simulink model "gm_MATE_HDLsolver_myFirstCircuit"  (R2024b)
settings: Solver=FixedStepDiscrete  StartTime=0.0  StopTime=0.05  FixedStep=6.02409638554217e-09  MaxStep=100e-6  RelTol=1e-4
PostLoadFcn:
  | Ts=1e-6; nb_sw=3; nb_lc=2;nb_r=1;nb_src=1; nb_out=3; rL=1.2;rC=100;L=1e-3; C=1e-5; LpejoSw=1e-6;h=Ts; MAX_INPUTS=16;
  | MAX_OUTPUTS=16;
  | MAX_SWITCHES=8;
  | MAX_INPUTS=16;
InitFcn:
  | Ts=1e-6; nb_sw=3; nb_lc=2;nb_r=1;nb_src=1; nb_out=3; rL=1.2;rC=100;L=1e-3; C=1e-5; LpejoSw=1e-6;h=Ts; MAX_INPUTS=16;
  | MAX_OUTPUTS=16;
  | MAX_SWITCHES=8;
  | MAX_INPUTS=16;
undefined symbols (not defined in the file or in its folder): MATE_SOC
libraries: fl_lib x31, nesl_utility x13, hdlmdlgenlib x10, simetranss x5, simulink x4, hdlsllib x3, ee_lib x2, eeGeneralControl x1
(part 5 of 8)

== system gm_MATE_HDLsolver_myFirstCircuit/ForFPGA/Dot Product79 ==
  In1 : Inport
  In2 : Inport  Port=2
  Dot Product79 : Sum  OutDataTypeStr=single  SampleTime=6.02409638554217e-09
  Dot Product79_pd1 : Delay  DelayLength=6
  Out1 : Outport
  wires:
  In1/1 -> Dot Product79/1
  In2/1 -> Dot Product79/2
  Dot Product79/1 -> Dot Product79_pd1/1
  Dot Product79_pd1/1 -> Out1/1

== system gm_MATE_HDLsolver_myFirstCircuit/ForFPGA/Dot Product8 ==
  In1 : Inport
  In2 : Inport  Port=2
  Dot Product8 : Sum  OutDataTypeStr=single  SampleTime=6.02409638554217e-09
  Dot Product8_pd1 : Delay  DelayLength=6
  Out1 : Outport
  wires:
  In1/1 -> Dot Product8/1
  In2/1 -> Dot Product8/2
  Dot Product8/1 -> Dot Product8_pd1/1
  Dot Product8_pd1/1 -> Out1/1

== system gm_MATE_HDLsolver_myFirstCircuit/ForFPGA/Dot Product81 ==
  In1 : Inport
  In2 : Inport  Port=2
  Dot Product81 : Sum  OutDataTypeStr=single  SampleTime=6.02409638554217e-09
  Dot Product81_pd1 : Delay  DelayLength=6
  Out1 : Outport
  wires:
  In1/1 -> Dot Product81/1
  In2/1 -> Dot Product81/2
  Dot Product81/1 -> Dot Product81_pd1/1
  Dot Product81_pd1/1 -> Out1/1

== system gm_MATE_HDLsolver_myFirstCircuit/ForFPGA/Dot Product810 ==
  In1 : Inport
  In2 : Inport  Port=2
  Dot Product810 : Sum  OutDataTypeStr=single  SampleTime=6.02409638554217e-09
  Dot Product810_pd1 : Delay  DelayLength=6
  Out1 : Outport
  wires:
  In1/1 -> Dot Product810/1
  In2/1 -> Dot Product810/2
  Dot Product810/1 -> Dot Product810_pd1/1
  Dot Product810_pd1/1 -> Out1/1

== system gm_MATE_HDLsolver_myFirstCircuit/ForFPGA/Dot Product811 ==
  In1 : Inport
  In2 : Inport  Port=2
  Dot Product811 : Sum  OutDataTypeStr=single  SampleTime=6.02409638554217e-09
  Dot Product811_pd1 : Delay  DelayLength=6
  Out1 : Outport
  wires:
  In1/1 -> Dot Product811/1
  In2/1 -> Dot Product811/2
  Dot Product811/1 -> Dot Product811_pd1/1
  Dot Product811_pd1/1 -> Out1/1

== system gm_MATE_HDLsolver_myFirstCircuit/ForFPGA/Dot Product812 ==
  In1 : Inport
  In2 : Inport  Port=2
  Dot Product812 : Sum  OutDataTypeStr=single  SampleTime=6.02409638554217e-09
  Dot Product812_pd1 : Delay  DelayLength=6
  Out1 : Outport
  wires:
  In1/1 -> Dot Product812/1
  In2/1 -> Dot Product812/2
  Dot Product812/1 -> Dot Product812_pd1/1
  Dot Product812_pd1/1 -> Out1/1

== system gm_MATE_HDLsolver_myFirstCircuit/ForFPGA/Dot Product813 ==
  In1 : Inport
  In2 : Inport  Port=2
  Dot Product813 : Sum  OutDataTypeStr=single  SampleTime=6.02409638554217e-09
  Dot Product813_pd1 : Delay  DelayLength=6
  Out1 : Outport
  wires:
  In1/1 -> Dot Product813/1
  In2/1 -> Dot Product813/2
  Dot Product813/1 -> Dot Product813_pd1/1
  Dot Product813_pd1/1 -> Out1/1

== system gm_MATE_HDLsolver_myFirstCircuit/ForFPGA/Dot Product814 ==
  In1 : Inport
  In2 : Inport  Port=2
  Dot Product814 : Sum  OutDataTypeStr=single  SampleTime=6.02409638554217e-09
  Dot Product814_pd1 : Delay  DelayLength=6
  Out1 : Outport
  wires:
  In1/1 -> Dot Product814/1
  In2/1 -> Dot Product814/2
  Dot Product814/1 -> Dot Product814_pd1/1
  Dot Product814_pd1/1 -> Out1/1

== system gm_MATE_HDLsolver_myFirstCircuit/ForFPGA/Dot Product815 ==
  In1 : Inport
  In2 : Inport  Port=2
  Dot Product815 : Sum  OutDataTypeStr=single  SampleTime=6.02409638554217e-09
  Dot Product815_pd1 : Delay  DelayLength=6
  Out1 : Outport
  wires:
  In1/1 -> Dot Product815/1
  In2/1 -> Dot Product815/2
  Dot Product815/1 -> Dot Product815_pd1/1
  Dot Product815_pd1/1 -> Out1/1

== system gm_MATE_HDLsolver_myFirstCircuit/ForFPGA/Dot Product82 ==
  In1 : Inport
  In2 : Inport  Port=2
  Dot Product82 : Sum  OutDataTypeStr=single  SampleTime=6.02409638554217e-09
  Dot Product82_pd1 : Delay  DelayLength=6
  Out1 : Outport
  wires:
  In1/1 -> Dot Product82/1
  In2/1 -> Dot Product82/2
  Dot Product82/1 -> Dot Product82_pd1/1
  Dot Product82_pd1/1 -> Out1/1

== system gm_MATE_HDLsolver_myFirstCircuit/ForFPGA/Dot Product83 ==
  In1 : Inport
  In2 : Inport  Port=2
  Dot Product83 : Sum  OutDataTypeStr=single  SampleTime=6.02409638554217e-09
  Dot Product83_pd1 : Delay  DelayLength=6
  Out1 : Outport
  wires:
  In1/1 -> Dot Product83/1
  In2/1 -> Dot Product83/2
  Dot Product83/1 -> Dot Product83_pd1/1
  Dot Product83_pd1/1 -> Out1/1

== system gm_MATE_HDLsolver_myFirstCircuit/ForFPGA/Dot Product84 ==
  In1 : Inport
  In2 : Inport  Port=2
  Dot Product84 : Sum  OutDataTypeStr=single  SampleTime=6.02409638554217e-09
  Dot Product84_pd1 : Delay  DelayLength=6
  Out1 : Outport
  wires:
  In1/1 -> Dot Product84/1
  In2/1 -> Dot Product84/2
  Dot Product84/1 -> Dot Product84_pd1/1
  Dot Product84_pd1/1 -> Out1/1

== system gm_MATE_HDLsolver_myFirstCircuit/ForFPGA/Dot Product85 ==
  In1 : Inport
  In2 : Inport  Port=2
  Dot Product85 : Sum  OutDataTypeStr=single  SampleTime=6.02409638554217e-09
  Dot Product85_pd1 : Delay  DelayLength=6
  Out1 : Outport
  wires:
  In1/1 -> Dot Product85/1
  In2/1 -> Dot Product85/2
  Dot Product85/1 -> Dot Product85_pd1/1
  Dot Product85_pd1/1 -> Out1/1

== system gm_MATE_HDLsolver_myFirstCircuit/ForFPGA/Dot Product86 ==
  In1 : Inport
  In2 : Inport  Port=2
  Dot Product86 : Sum  OutDataTypeStr=single  SampleTime=6.02409638554217e-09
  Dot Product86_pd1 : Delay  DelayLength=6
  Out1 : Outport
  wires:
  In1/1 -> Dot Product86/1
  In2/1 -> Dot Product86/2
  Dot Product86/1 -> Dot Product86_pd1/1
  Dot Product86_pd1/1 -> Out1/1

== system gm_MATE_HDLsolver_myFirstCircuit/ForFPGA/Dot Product87 ==
  In1 : Inport
  In2 : Inport  Port=2
  Dot Product87 : Sum  OutDataTypeStr=single  SampleTime=6.02409638554217e-09
  Dot Product87_pd1 : Delay  DelayLength=6
  Out1 : Outport
  wires:
  In1/1 -> Dot Product87/1
  In2/1 -> Dot Product87/2
  Dot Product87/1 -> Dot Product87_pd1/1
  Dot Product87_pd1/1 -> Out1/1

== system gm_MATE_HDLsolver_myFirstCircuit/ForFPGA/Dot Product88 ==
  In1 : Inport
  In2 : Inport  Port=2
  Dot Product88 : Sum  OutDataTypeStr=single  SampleTime=6.02409638554217e-09
  Dot Product88_pd1 : Delay  DelayLength=6
  Out1 : Outport
  wires:
  In1/1 -> Dot Product88/1
  In2/1 -> Dot Product88/2
  Dot Product88/1 -> Dot Product88_pd1/1
  Dot Product88_pd1/1 -> Out1/1

== system gm_MATE_HDLsolver_myFirstCircuit/ForFPGA/Dot Product89 ==
  In1 : Inport
  In2 : Inport  Port=2
  Dot Product89 : Sum  OutDataTypeStr=single  SampleTime=6.02409638554217e-09
  Dot Product89_pd1 : Delay  DelayLength=6
  Out1 : Outport
  wires:
  In1/1 -> Dot Product89/1
  In2/1 -> Dot Product89/2
  Dot Product89/1 -> Dot Product89_pd1/1
  Dot Product89_pd1/1 -> Out1/1

== system gm_MATE_HDLsolver_myFirstCircuit/ForFPGA/Dot Product9 ==
  In1 : Inport
  In2 : Inport  Port=2
  Dot Product9 : Sum  OutDataTypeStr=single  SampleTime=6.02409638554217e-09
  Dot Product9_pd1 : Delay  DelayLength=6
  Out1 : Outport
  wires:
  In1/1 -> Dot Product9/1
  In2/1 -> Dot Product9/2
  Dot Product9/1 -> Dot Product9_pd1/1
  Dot Product9_pd1/1 -> Out1/1

== system gm_MATE_HDLsolver_myFirstCircuit/ForFPGA/Dot Product91 ==
  In1 : Inport
  In2 : Inport  Port=2
  Dot Product91 : Sum  OutDataTypeStr=single  SampleTime=6.02409638554217e-09
  Dot Product91_pd1 : Delay  DelayLength=6
  Out1 : Outport
  wires:
  In1/1 -> Dot Product91/1
  In2/1 -> Dot Product91/2
  Dot Product91/1 -> Dot Product91_pd1/1
  Dot Product91_pd1/1 -> Out1/1

== system gm_MATE_HDLsolver_myFirstCircuit/ForFPGA/Dot Product910 ==
  In1 : Inport
  In2 : Inport  Port=2
  Dot Product910 : Sum  OutDataTypeStr=single  SampleTime=6.02409638554217e-09
  Dot Product910_pd1 : Delay  DelayLength=6
  Out1 : Outport
  wires:
  In1/1 -> Dot Product910/1
  In2/1 -> Dot Product910/2
  Dot Product910/1 -> Dot Product910_pd1/1
  Dot Product910_pd1/1 -> Out1/1

== system gm_MATE_HDLsolver_myFirstCircuit/ForFPGA/Dot Product911 ==
  In1 : Inport
  In2 : Inport  Port=2
  Dot Product911 : Sum  OutDataTypeStr=single  SampleTime=6.02409638554217e-09
  Dot Product911_pd1 : Delay  DelayLength=6
  Out1 : Outport
  wires:
  In1/1 -> Dot Product911/1
  In2/1 -> Dot Product911/2
  Dot Product911/1 -> Dot Product911_pd1/1
  Dot Product911_pd1/1 -> Out1/1

== system gm_MATE_HDLsolver_myFirstCircuit/ForFPGA/Dot Product912 ==
  In1 : Inport
  In2 : Inport  Port=2
  Dot Product912 : Sum  OutDataTypeStr=single  SampleTime=6.02409638554217e-09
  Dot Product912_pd1 : Delay  DelayLength=6
  Out1 : Outport
  wires:
  In1/1 -> Dot Product912/1
  In2/1 -> Dot Product912/2
  Dot Product912/1 -> Dot Product912_pd1/1
  Dot Product912_pd1/1 -> Out1/1

== system gm_MATE_HDLsolver_myFirstCircuit/ForFPGA/Dot Product913 ==
  In1 : Inport
  In2 : Inport  Port=2
  Dot Product913 : Sum  OutDataTypeStr=single  SampleTime=6.02409638554217e-09
  Dot Product913_pd1 : Delay  DelayLength=6
  Out1 : Outport
  wires:
  In1/1 -> Dot Product913/1
  In2/1 -> Dot Product913/2
  Dot Product913/1 -> Dot Product913_pd1/1
  Dot Product913_pd1/1 -> Out1/1

== system gm_MATE_HDLsolver_myFirstCircuit/ForFPGA/Dot Product914 ==
  In1 : Inport
  In2 : Inport  Port=2
  Dot Product914 : Sum  OutDataTypeStr=single  SampleTime=6.02409638554217e-09
  Dot Product914_pd1 : Delay  DelayLength=6
  Out1 : Outport
  wires:
  In1/1 -> Dot Product914/1
  In2/1 -> Dot Product914/2
  Dot Product914/1 -> Dot Product914_pd1/1
  Dot Product914_pd1/1 -> Out1/1

== system gm_MATE_HDLsolver_myFirstCircuit/ForFPGA/Dot Product915 ==
  In1 : Inport
  In2 : Inport  Port=2
  Dot Product915 : Sum  OutDataTypeStr=single  SampleTime=6.02409638554217e-09
  Dot Product915_pd1 : Delay  DelayLength=6
  Out1 : Outport
  wires:
  In1/1 -> Dot Product915/1
  In2/1 -> Dot Product915/2
  Dot Product915/1 -> Dot Product915_pd1/1
  Dot Product915_pd1/1 -> Out1/1

== system gm_MATE_HDLsolver_myFirstCircuit/ForFPGA/Dot Product92 ==
  In1 : Inport
  In2 : Inport  Port=2
  Dot Product92 : Sum  OutDataTypeStr=single  SampleTime=6.02409638554217e-09
  Dot Product92_pd1 : Delay  DelayLength=6
  Out1 : Outport
  wires:
  In1/1 -> Dot Product92/1
  In2/1 -> Dot Product92/2
  Dot Product92/1 -> Dot Product92_pd1/1
  Dot Product92_pd1/1 -> Out1/1

== system gm_MATE_HDLsolver_myFirstCircuit/ForFPGA/Dot Product93 ==
  In1 : Inport
  In2 : Inport  Port=2
  Dot Product93 : Sum  OutDataTypeStr=single  SampleTime=6.02409638554217e-09
  Dot Product93_pd1 : Delay  DelayLength=6
  Out1 : Outport
  wires:
  In1/1 -> Dot Product93/1
  In2/1 -> Dot Product93/2
  Dot Product93/1 -> Dot Product93_pd1/1
  Dot Product93_pd1/1 -> Out1/1

== system gm_MATE_HDLsolver_myFirstCircuit/ForFPGA/Dot Product94 ==
  In1 : Inport
  In2 : Inport  Port=2
  Dot Product94 : Sum  OutDataTypeStr=single  SampleTime=6.02409638554217e-09
  Dot Product94_pd1 : Delay  DelayLength=6
  Out1 : Outport
  wires:
  In1/1 -> Dot Product94/1
  In2/1 -> Dot Product94/2
  Dot Product94/1 -> Dot Product94_pd1/1
  Dot Product94_pd1/1 -> Out1/1

== system gm_MATE_HDLsolver_myFirstCircuit/ForFPGA/Dot Product95 ==
  In1 : Inport
  In2 : Inport  Port=2
  Dot Product95 : Sum  OutDataTypeStr=single  SampleTime=6.02409638554217e-09
  Dot Product95_pd1 : Delay  DelayLength=6
  Out1 : Outport
  wires:
  In1/1 -> Dot Product95/1
  In2/1 -> Dot Product95/2
  Dot Product95/1 -> Dot Product95_pd1/1
  Dot Product95_pd1/1 -> Out1/1

== system gm_MATE_HDLsolver_myFirstCircuit/ForFPGA/Dot Product96 ==
  In1 : Inport
  In2 : Inport  Port=2
  Dot Product96 : Sum  OutDataTypeStr=single  SampleTime=6.02409638554217e-09
  Dot Product96_pd1 : Delay  DelayLength=6
  Out1 : Outport
  wires:
  In1/1 -> Dot Product96/1
  In2/1 -> Dot Product96/2
  Dot Product96/1 -> Dot Product96_pd1/1
  Dot Product96_pd1/1 -> Out1/1

== system gm_MATE_HDLsolver_myFirstCircuit/ForFPGA/Dot Product97 ==
  In1 : Inport
  In2 : Inport  Port=2
  Dot Product97 : Sum  OutDataTypeStr=single  SampleTime=6.02409638554217e-09
  Dot Product97_pd1 : Delay  DelayLength=6
  Out1 : Outport
  wires:
  In1/1 -> Dot Product97/1
  In2/1 -> Dot Product97/2
  Dot Product97/1 -> Dot Product97_pd1/1
  Dot Product97_pd1/1 -> Out1/1

== system gm_MATE_HDLsolver_myFirstCircuit/ForFPGA/Dot Product98 ==
  In1 : Inport
  In2 : Inport  Port=2
  Dot Product98 : Sum  OutDataTypeStr=single  SampleTime=6.02409638554217e-09
  Dot Product98_pd1 : Delay  DelayLength=6
  Out1 : Outport
  wires:
  In1/1 -> Dot Product98/1
  In2/1 -> Dot Product98/2
  Dot Product98/1 -> Dot Product98_pd1/1
  Dot Product98_pd1/1 -> Out1/1

== system gm_MATE_HDLsolver_myFirstCircuit/ForFPGA/Dot Product99 ==
  In1 : Inport
  In2 : Inport  Port=2
  Dot Product99 : Sum  OutDataTypeStr=single  SampleTime=6.02409638554217e-09
  Dot Product99_pd1 : Delay  DelayLength=6
  Out1 : Outport
  wires:
  In1/1 -> Dot Product99/1
  In2/1 -> Dot Product99/2
  Dot Product99/1 -> Dot Product99_pd1/1
  Dot Product99_pd1/1 -> Out1/1

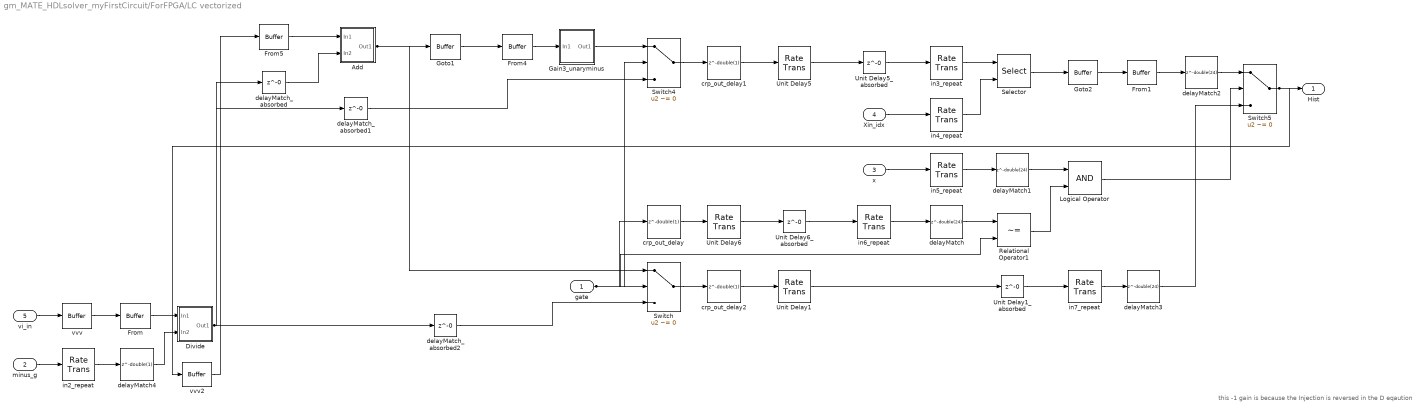
== system gm_MATE_HDLsolver_myFirstCircuit/ForFPGA/LC vectorized ==
  note: this -1 gain is because the Injection is reversed in the D eqaution
  gate : Inport  OutDataTypeStr=boolean  PortDimensions=[5]  SampleTime=6.02409638554217e-09
  minus_g : Inport  Port=2  OutDataTypeStr=single  PortDimensions=[5]  SampleTime=1e-06
  x : Inport  Port=3  OutDataTypeStr=boolean  PortDimensions=[5]  SampleTime=1e-06
  Xin_idx : Inport  Port=4  OutDataTypeStr=uint16  PortDimensions=[5]  SampleTime=1e-06
  vi_in : Inport  Port=5  OutDataTypeStr=single  PortDimensions=[5]  SampleTime=6.02409638554217e-09
  Add : Subsystem
      mask Display: disp('NFP\nadd');
  Divide : Subsystem
      mask Display: disp('NFP\nmul');
  From{,1,4..5} (4 alike) : hdlmdlgenlib/Buffer
  Gain3_unaryminus : Subsystem
      mask Display: disp('NFP\numinus');
  Goto1 : hdlmdlgenlib/Buffer
  Goto2 : hdlmdlgenlib/Buffer
  Logical Operator : Logic  AllPortsSameDT=off  OutDataTypeStr=boolean  SampleTime=6.02409638554217e-09
  Relational Operator1 : RelationalOperator  Operator=~=  OutDataTypeStr=boolean  SampleTime=6.02409638554217e-09  InputSameDT=off
  Selector : Selector  InputPortWidth=5  IndexOptions=Index vector (port)  Indices=double([2 1 3 4 5])  OutputSizes=double(1)
  Switch : Switch  Criteria=u2 ~= 0  Threshold=double(0)  OutDataTypeStr=single  SampleTime=6.02409638554217e-09  SaturateOnIntegerOverflow=off  InputSameDT=off
  Switch4 : Switch  Criteria=u2 ~= 0  Threshold=double(0)  OutDataTypeStr=single  SampleTime=6.02409638554217e-09  SaturateOnIntegerOverflow=off  InputSameDT=off
  Switch5 : Switch  Criteria=u2 ~= 0  Threshold=double(0)  OutDataTypeStr=single  SampleTime=6.02409638554217e-09  SaturateOnIntegerOverflow=off  InputSameDT=off
  Unit Delay1 : RateTransition  InitialCondition=double(0)  OutPortSampleTimeOpt=Multiple of input port sample time  OutPortSampleTimeMultiple=166
  Unit Delay1_absorbed : Delay  DelayLength=0
  Unit Delay5 : RateTransition  InitialCondition=double(0)  OutPortSampleTimeOpt=Multiple of input port sample time  OutPortSampleTimeMultiple=166
  Unit Delay5_absorbed : Delay  DelayLength=0
  Unit Delay6 : RateTransition  InitialCondition=double(0)  OutPortSampleTimeOpt=Multiple of input port sample time  OutPortSampleTimeMultiple=166
  Unit Delay6_absorbed : Delay  DelayLength=0
  crp_out_delay : Delay  DelayLength=double(1)  InitialCondition=0  SampleTime=6.02409638554217e-09
  crp_out_delay1 : Delay  DelayLength=double(1)  InitialCondition=0  SampleTime=6.02409638554217e-09
  crp_out_delay2 : Delay  DelayLength=double(1)  InitialCondition=0  SampleTime=6.02409638554217e-09
  delayMatch{,1..3} (4 alike) : Delay  DelayLength=double(24)  InitialCondition=0  SampleTime=6.02409638554217e-09
  delayMatch4 : Delay  DelayLength=double(1)  InitialCondition=0  SampleTime=6.02409638554217e-09
  delayMatch_absorbed : Delay  DelayLength=0
  delayMatch_absorbed1 : Delay  DelayLength=0
  delayMatch_absorbed2 : Delay  DelayLength=0
  in2_repeat : RateTransition  Integrity=off  Deterministic=off  OutPortSampleTimeOpt=Multiple of input port sample time  OutPortSampleTimeMultiple=1/166
  in3_repeat : RateTransition  Integrity=off  Deterministic=off  OutPortSampleTimeOpt=Multiple of input port sample time  OutPortSampleTimeMultiple=1/166
  in4_repeat : RateTransition  Integrity=off  Deterministic=off  OutPortSampleTimeOpt=Multiple of input port sample time  OutPortSampleTimeMultiple=1/166
  in5_repeat : RateTransition  Integrity=off  Deterministic=off  OutPortSampleTimeOpt=Multiple of input port sample time  OutPortSampleTimeMultiple=1/166
  in6_repeat : RateTransition  Integrity=off  Deterministic=off  OutPortSampleTimeOpt=Multiple of input port sample time  OutPortSampleTimeMultiple=1/166
  in7_repeat : RateTransition  Integrity=off  Deterministic=off  OutPortSampleTimeOpt=Multiple of input port sample time  OutPortSampleTimeMultiple=1/166
  vvv : hdlmdlgenlib/Buffer
  vvv2 : hdlmdlgenlib/Buffer
  Hist : Outport  SampleTime=6.02409638554217e-09
  wires:
  delayMatch4/1 -> Divide/2(In2)
  in7_repeat/1 -> delayMatch3/1
  vi_in/1 -> vvv/1
  Logical Operator/1 -> Switch5/2
  minus_g/1 -> in2_repeat/1
  vvv2/1 -> From5/1
  Unit Delay1/1 -> Unit Delay1_absorbed/1
  in2_repeat/1 -> delayMatch4/1
  delayMatch_absorbed2/1 -> Switch/3
  Divide/1(Out1) -> delayMatch_absorbed1/1, delayMatch_absorbed2/1, delayMatch_absorbed/1
  vvv/1 -> From/1
  From/1 -> Divide/1(In1)
  From5/1 -> Add/1(In1)
  delayMatch_absorbed/1 -> Add/2(In2)
  Add/1(Out1) -> Goto1/1, Switch/1
  crp_out_delay1/1 -> Unit Delay5/1
  delayMatch_absorbed1/1 -> Switch4/3
  Goto1/1 -> From4/1
  From4/1 -> Gain3_unaryminus/1(In1)
  Gain3_unaryminus/1(Out1) -> Switch4/1
  Unit Delay6/1 -> Unit Delay6_absorbed/1
  gate/1 -> Relational Operator1/2, crp_out_delay/1, Switch/2, Switch4/2
  Switch4/1 -> crp_out_delay1/1
  in4_repeat/1 -> Selector/2
  crp_out_delay/1 -> Unit Delay6/1
  Xin_idx/1 -> in4_repeat/1
  Switch/1 -> crp_out_delay2/1
  crp_out_delay2/1 -> Unit Delay1/1
  Unit Delay5/1 -> Unit Delay5_absorbed/1
  Unit Delay1_absorbed/1 -> in7_repeat/1
  Unit Delay6_absorbed/1 -> in6_repeat/1
  Unit Delay5_absorbed/1 -> in3_repeat/1
  Switch5/1 -> Hist/1, vvv2/1
  x/1 -> in5_repeat/1
  in6_repeat/1 -> delayMatch/1
  in3_repeat/1 -> Selector/1
  in5_repeat/1 -> delayMatch1/1
  delayMatch/1 -> Relational Operator1/1
  Selector/1 -> Goto2/1
  delayMatch3/1 -> Switch5/3
  delayMatch1/1 -> Logical Operator/1
  Relational Operator1/1 -> Logical Operator/2
  Goto2/1 -> From1/1
  From1/1 -> delayMatch2/1
  delayMatch2/1 -> Switch5/1

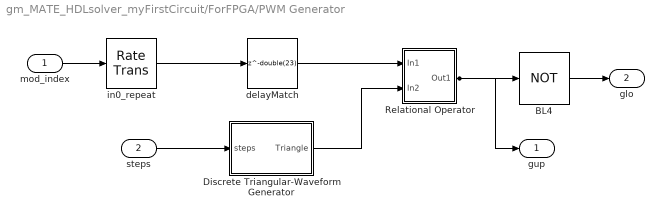
== system gm_MATE_HDLsolver_myFirstCircuit/ForFPGA/PWM Generator ==
  mod_index : Inport  OutDataTypeStr=single  PortDimensions=1  SampleTime=1e-06
  steps : Inport  Port=2  OutDataTypeStr=uint16  PortDimensions=1  SampleTime=1e-06
  BL4 : Logic  Operator=NOT  Inputs=1  AllPortsSameDT=off  OutDataTypeStr=boolean  SampleTime=6.02409638554217e-09
  Discrete Triangular-Waveform Generator : Subsystem
  Relational Operator : Subsystem
      mask Display: disp('NFP\nrelop');
  delayMatch : Delay  DelayLength=double(23)  InitialCondition=0  SampleTime=6.02409638554217e-09
  in0_repeat : RateTransition  Integrity=off  Deterministic=off  OutPortSampleTimeOpt=Multiple of input port sample time  OutPortSampleTimeMultiple=1/166
  gup : Outport  SampleTime=6.02409638554217e-09  VectorParamsAs1DForOutWhenUnconnected=off
  glo : Outport  Port=2  SampleTime=6.02409638554217e-09  VectorParamsAs1DForOutWhenUnconnected=off
  wires:
  Relational Operator/1(Out1) -> gup/1, BL4/1
  mod_index/1 -> in0_repeat/1
  delayMatch/1 -> Relational Operator/1(In1)
  in0_repeat/1 -> delayMatch/1
  steps/1 -> Discrete Triangular-Waveform Generator/1(steps)
  Discrete Triangular-Waveform Generator/1(Triangle) -> Relational Operator/2(In2)
  BL4/1 -> glo/1

== system gm_MATE_HDLsolver_myFirstCircuit/ForFPGA/mul_Dot Product10_dotp_0 ==
  In1 : Inport
  In2 : Inport  Port=2
  mul_Dot Product10_dotp_0 : Product  Inputs=**  OutDataTypeStr=single  SampleTime=6.02409638554217e-09
  mul_Dot Product10_dotp_0_pd1 : Delay  DelayLength=6
  Out1 : Outport
  wires:
  In1/1 -> mul_Dot Product10_dotp_0/1
  In2/1 -> mul_Dot Product10_dotp_0/2
  mul_Dot Product10_dotp_0/1 -> mul_Dot Product10_dotp_0_pd1/1
  mul_Dot Product10_dotp_0_pd1/1 -> Out1/1

== system gm_MATE_HDLsolver_myFirstCircuit/ForFPGA/mul_Dot Product10_dotp_1 ==
  In1 : Inport
  In2 : Inport  Port=2
  mul_Dot Product10_dotp_1 : Product  Inputs=**  OutDataTypeStr=single  SampleTime=6.02409638554217e-09
  mul_Dot Product10_dotp_1_pd1 : Delay  DelayLength=6
  Out1 : Outport
  wires:
  In1/1 -> mul_Dot Product10_dotp_1/1
  In2/1 -> mul_Dot Product10_dotp_1/2
  mul_Dot Product10_dotp_1/1 -> mul_Dot Product10_dotp_1_pd1/1
  mul_Dot Product10_dotp_1_pd1/1 -> Out1/1

== system gm_MATE_HDLsolver_myFirstCircuit/ForFPGA/mul_Dot Product10_dotp_10 ==
  In1 : Inport
  In2 : Inport  Port=2
  mul_Dot Product10_dotp_10 : Product  Inputs=**  OutDataTypeStr=single  SampleTime=6.02409638554217e-09
  mul_Dot Product10_dotp_10_pd1 : Delay  DelayLength=6
  Out1 : Outport
  wires:
  In1/1 -> mul_Dot Product10_dotp_10/1
  In2/1 -> mul_Dot Product10_dotp_10/2
  mul_Dot Product10_dotp_10/1 -> mul_Dot Product10_dotp_10_pd1/1
  mul_Dot Product10_dotp_10_pd1/1 -> Out1/1

== system gm_MATE_HDLsolver_myFirstCircuit/ForFPGA/mul_Dot Product10_dotp_11 ==
  In1 : Inport
  In2 : Inport  Port=2
  mul_Dot Product10_dotp_11 : Product  Inputs=**  OutDataTypeStr=single  SampleTime=6.02409638554217e-09
  mul_Dot Product10_dotp_11_pd1 : Delay  DelayLength=6
  Out1 : Outport
  wires:
  In1/1 -> mul_Dot Product10_dotp_11/1
  In2/1 -> mul_Dot Product10_dotp_11/2
  mul_Dot Product10_dotp_11/1 -> mul_Dot Product10_dotp_11_pd1/1
  mul_Dot Product10_dotp_11_pd1/1 -> Out1/1

== system gm_MATE_HDLsolver_myFirstCircuit/ForFPGA/mul_Dot Product10_dotp_12 ==
  In1 : Inport
  In2 : Inport  Port=2
  mul_Dot Product10_dotp_12 : Product  Inputs=**  OutDataTypeStr=single  SampleTime=6.02409638554217e-09
  mul_Dot Product10_dotp_12_pd1 : Delay  DelayLength=6
  Out1 : Outport
  wires:
  In1/1 -> mul_Dot Product10_dotp_12/1
  In2/1 -> mul_Dot Product10_dotp_12/2
  mul_Dot Product10_dotp_12/1 -> mul_Dot Product10_dotp_12_pd1/1
  mul_Dot Product10_dotp_12_pd1/1 -> Out1/1

== system gm_MATE_HDLsolver_myFirstCircuit/ForFPGA/mul_Dot Product10_dotp_13 ==
  In1 : Inport
  In2 : Inport  Port=2
  mul_Dot Product10_dotp_13 : Product  Inputs=**  OutDataTypeStr=single  SampleTime=6.02409638554217e-09
  mul_Dot Product10_dotp_13_pd1 : Delay  DelayLength=6
  Out1 : Outport
  wires:
  In1/1 -> mul_Dot Product10_dotp_13/1
  In2/1 -> mul_Dot Product10_dotp_13/2
  mul_Dot Product10_dotp_13/1 -> mul_Dot Product10_dotp_13_pd1/1
  mul_Dot Product10_dotp_13_pd1/1 -> Out1/1

== system gm_MATE_HDLsolver_myFirstCircuit/ForFPGA/mul_Dot Product10_dotp_14 ==
  In1 : Inport
  In2 : Inport  Port=2
  mul_Dot Product10_dotp_14 : Product  Inputs=**  OutDataTypeStr=single  SampleTime=6.02409638554217e-09
  mul_Dot Product10_dotp_14_pd1 : Delay  DelayLength=6
  Out1 : Outport
  wires:
  In1/1 -> mul_Dot Product10_dotp_14/1
  In2/1 -> mul_Dot Product10_dotp_14/2
  mul_Dot Product10_dotp_14/1 -> mul_Dot Product10_dotp_14_pd1/1
  mul_Dot Product10_dotp_14_pd1/1 -> Out1/1

== system gm_MATE_HDLsolver_myFirstCircuit/ForFPGA/mul_Dot Product10_dotp_15 ==
  In1 : Inport
  In2 : Inport  Port=2
  mul_Dot Product10_dotp_15 : Product  Inputs=**  OutDataTypeStr=single  SampleTime=6.02409638554217e-09
  mul_Dot Product10_dotp_15_pd1 : Delay  DelayLength=6
  Out1 : Outport
  wires:
  In1/1 -> mul_Dot Product10_dotp_15/1
  In2/1 -> mul_Dot Product10_dotp_15/2
  mul_Dot Product10_dotp_15/1 -> mul_Dot Product10_dotp_15_pd1/1
  mul_Dot Product10_dotp_15_pd1/1 -> Out1/1

== system gm_MATE_HDLsolver_myFirstCircuit/ForFPGA/mul_Dot Product10_dotp_2 ==
  In1 : Inport
  In2 : Inport  Port=2
  mul_Dot Product10_dotp_2 : Product  Inputs=**  OutDataTypeStr=single  SampleTime=6.02409638554217e-09
  mul_Dot Product10_dotp_2_pd1 : Delay  DelayLength=6
  Out1 : Outport
  wires:
  In1/1 -> mul_Dot Product10_dotp_2/1
  In2/1 -> mul_Dot Product10_dotp_2/2
  mul_Dot Product10_dotp_2/1 -> mul_Dot Product10_dotp_2_pd1/1
  mul_Dot Product10_dotp_2_pd1/1 -> Out1/1

== system gm_MATE_HDLsolver_myFirstCircuit/ForFPGA/mul_Dot Product10_dotp_3 ==
  In1 : Inport
  In2 : Inport  Port=2
  mul_Dot Product10_dotp_3 : Product  Inputs=**  OutDataTypeStr=single  SampleTime=6.02409638554217e-09
  mul_Dot Product10_dotp_3_pd1 : Delay  DelayLength=6
  Out1 : Outport
  wires:
  In1/1 -> mul_Dot Product10_dotp_3/1
  In2/1 -> mul_Dot Product10_dotp_3/2
  mul_Dot Product10_dotp_3/1 -> mul_Dot Product10_dotp_3_pd1/1
  mul_Dot Product10_dotp_3_pd1/1 -> Out1/1

== system gm_MATE_HDLsolver_myFirstCircuit/ForFPGA/mul_Dot Product10_dotp_4 ==
  In1 : Inport
  In2 : Inport  Port=2
  mul_Dot Product10_dotp_4 : Product  Inputs=**  OutDataTypeStr=single  SampleTime=6.02409638554217e-09
  mul_Dot Product10_dotp_4_pd1 : Delay  DelayLength=6
  Out1 : Outport
  wires:
  In1/1 -> mul_Dot Product10_dotp_4/1
  In2/1 -> mul_Dot Product10_dotp_4/2
  mul_Dot Product10_dotp_4/1 -> mul_Dot Product10_dotp_4_pd1/1
  mul_Dot Product10_dotp_4_pd1/1 -> Out1/1

== system gm_MATE_HDLsolver_myFirstCircuit/ForFPGA/mul_Dot Product10_dotp_5 ==
  In1 : Inport
  In2 : Inport  Port=2
  mul_Dot Product10_dotp_5 : Product  Inputs=**  OutDataTypeStr=single  SampleTime=6.02409638554217e-09
  mul_Dot Product10_dotp_5_pd1 : Delay  DelayLength=6
  Out1 : Outport
  wires:
  In1/1 -> mul_Dot Product10_dotp_5/1
  In2/1 -> mul_Dot Product10_dotp_5/2
  mul_Dot Product10_dotp_5/1 -> mul_Dot Product10_dotp_5_pd1/1
  mul_Dot Product10_dotp_5_pd1/1 -> Out1/1

== system gm_MATE_HDLsolver_myFirstCircuit/ForFPGA/mul_Dot Product10_dotp_6 ==
  In1 : Inport
  In2 : Inport  Port=2
  mul_Dot Product10_dotp_6 : Product  Inputs=**  OutDataTypeStr=single  SampleTime=6.02409638554217e-09
  mul_Dot Product10_dotp_6_pd1 : Delay  DelayLength=6
  Out1 : Outport
  wires:
  In1/1 -> mul_Dot Product10_dotp_6/1
  In2/1 -> mul_Dot Product10_dotp_6/2
  mul_Dot Product10_dotp_6/1 -> mul_Dot Product10_dotp_6_pd1/1
  mul_Dot Product10_dotp_6_pd1/1 -> Out1/1

== system gm_MATE_HDLsolver_myFirstCircuit/ForFPGA/mul_Dot Product10_dotp_7 ==
  In1 : Inport
  In2 : Inport  Port=2
  mul_Dot Product10_dotp_7 : Product  Inputs=**  OutDataTypeStr=single  SampleTime=6.02409638554217e-09
  mul_Dot Product10_dotp_7_pd1 : Delay  DelayLength=6
  Out1 : Outport
  wires:
  In1/1 -> mul_Dot Product10_dotp_7/1
  In2/1 -> mul_Dot Product10_dotp_7/2
  mul_Dot Product10_dotp_7/1 -> mul_Dot Product10_dotp_7_pd1/1
  mul_Dot Product10_dotp_7_pd1/1 -> Out1/1

== system gm_MATE_HDLsolver_myFirstCircuit/ForFPGA/mul_Dot Product10_dotp_8 ==
  In1 : Inport
  In2 : Inport  Port=2
  mul_Dot Product10_dotp_8 : Product  Inputs=**  OutDataTypeStr=single  SampleTime=6.02409638554217e-09
  mul_Dot Product10_dotp_8_pd1 : Delay  DelayLength=6
  Out1 : Outport
  wires:
  In1/1 -> mul_Dot Product10_dotp_8/1
  In2/1 -> mul_Dot Product10_dotp_8/2
  mul_Dot Product10_dotp_8/1 -> mul_Dot Product10_dotp_8_pd1/1
  mul_Dot Product10_dotp_8_pd1/1 -> Out1/1

== system gm_MATE_HDLsolver_myFirstCircuit/ForFPGA/mul_Dot Product10_dotp_9 ==
  In1 : Inport
  In2 : Inport  Port=2
  mul_Dot Product10_dotp_9 : Product  Inputs=**  OutDataTypeStr=single  SampleTime=6.02409638554217e-09
  mul_Dot Product10_dotp_9_pd1 : Delay  DelayLength=6
  Out1 : Outport
  wires:
  In1/1 -> mul_Dot Product10_dotp_9/1
  In2/1 -> mul_Dot Product10_dotp_9/2
  mul_Dot Product10_dotp_9/1 -> mul_Dot Product10_dotp_9_pd1/1
  mul_Dot Product10_dotp_9_pd1/1 -> Out1/1

== system gm_MATE_HDLsolver_myFirstCircuit/ForFPGA/mul_Dot Product11_dotp_0 ==
  In1 : Inport
  In2 : Inport  Port=2
  mul_Dot Product11_dotp_0 : Product  Inputs=**  OutDataTypeStr=single  SampleTime=6.02409638554217e-09
  mul_Dot Product11_dotp_0_pd1 : Delay  DelayLength=6
  Out1 : Outport
  wires:
  In1/1 -> mul_Dot Product11_dotp_0/1
  In2/1 -> mul_Dot Product11_dotp_0/2
  mul_Dot Product11_dotp_0/1 -> mul_Dot Product11_dotp_0_pd1/1
  mul_Dot Product11_dotp_0_pd1/1 -> Out1/1

== system gm_MATE_HDLsolver_myFirstCircuit/ForFPGA/mul_Dot Product11_dotp_1 ==
  In1 : Inport
  In2 : Inport  Port=2
  mul_Dot Product11_dotp_1 : Product  Inputs=**  OutDataTypeStr=single  SampleTime=6.02409638554217e-09
  mul_Dot Product11_dotp_1_pd1 : Delay  DelayLength=6
  Out1 : Outport
  wires:
  In1/1 -> mul_Dot Product11_dotp_1/1
  In2/1 -> mul_Dot Product11_dotp_1/2
  mul_Dot Product11_dotp_1/1 -> mul_Dot Product11_dotp_1_pd1/1
  mul_Dot Product11_dotp_1_pd1/1 -> Out1/1

== system gm_MATE_HDLsolver_myFirstCircuit/ForFPGA/mul_Dot Product11_dotp_10 ==
  In1 : Inport
  In2 : Inport  Port=2
  mul_Dot Product11_dotp_10 : Product  Inputs=**  OutDataTypeStr=single  SampleTime=6.02409638554217e-09
  mul_Dot Product11_dotp_10_pd1 : Delay  DelayLength=6
  Out1 : Outport
  wires:
  In1/1 -> mul_Dot Product11_dotp_10/1
  In2/1 -> mul_Dot Product11_dotp_10/2
  mul_Dot Product11_dotp_10/1 -> mul_Dot Product11_dotp_10_pd1/1
  mul_Dot Product11_dotp_10_pd1/1 -> Out1/1

== system gm_MATE_HDLsolver_myFirstCircuit/ForFPGA/mul_Dot Product11_dotp_11 ==
  In1 : Inport
  In2 : Inport  Port=2
  mul_Dot Product11_dotp_11 : Product  Inputs=**  OutDataTypeStr=single  SampleTime=6.02409638554217e-09
  mul_Dot Product11_dotp_11_pd1 : Delay  DelayLength=6
  Out1 : Outport
  wires:
  In1/1 -> mul_Dot Product11_dotp_11/1
  In2/1 -> mul_Dot Product11_dotp_11/2
  mul_Dot Product11_dotp_11/1 -> mul_Dot Product11_dotp_11_pd1/1
  mul_Dot Product11_dotp_11_pd1/1 -> Out1/1

== system gm_MATE_HDLsolver_myFirstCircuit/ForFPGA/mul_Dot Product11_dotp_12 ==
  In1 : Inport
  In2 : Inport  Port=2
  mul_Dot Product11_dotp_12 : Product  Inputs=**  OutDataTypeStr=single  SampleTime=6.02409638554217e-09
  mul_Dot Product11_dotp_12_pd1 : Delay  DelayLength=6
  Out1 : Outport
  wires:
  In1/1 -> mul_Dot Product11_dotp_12/1
  In2/1 -> mul_Dot Product11_dotp_12/2
  mul_Dot Product11_dotp_12/1 -> mul_Dot Product11_dotp_12_pd1/1
  mul_Dot Product11_dotp_12_pd1/1 -> Out1/1

== system gm_MATE_HDLsolver_myFirstCircuit/ForFPGA/mul_Dot Product11_dotp_13 ==
  In1 : Inport
  In2 : Inport  Port=2
  mul_Dot Product11_dotp_13 : Product  Inputs=**  OutDataTypeStr=single  SampleTime=6.02409638554217e-09
  mul_Dot Product11_dotp_13_pd1 : Delay  DelayLength=6
  Out1 : Outport
  wires:
  In1/1 -> mul_Dot Product11_dotp_13/1
  In2/1 -> mul_Dot Product11_dotp_13/2
  mul_Dot Product11_dotp_13/1 -> mul_Dot Product11_dotp_13_pd1/1
  mul_Dot Product11_dotp_13_pd1/1 -> Out1/1

== system gm_MATE_HDLsolver_myFirstCircuit/ForFPGA/mul_Dot Product11_dotp_14 ==
  In1 : Inport
  In2 : Inport  Port=2
  mul_Dot Product11_dotp_14 : Product  Inputs=**  OutDataTypeStr=single  SampleTime=6.02409638554217e-09
  mul_Dot Product11_dotp_14_pd1 : Delay  DelayLength=6
  Out1 : Outport
  wires:
  In1/1 -> mul_Dot Product11_dotp_14/1
  In2/1 -> mul_Dot Product11_dotp_14/2
  mul_Dot Product11_dotp_14/1 -> mul_Dot Product11_dotp_14_pd1/1
  mul_Dot Product11_dotp_14_pd1/1 -> Out1/1

== system gm_MATE_HDLsolver_myFirstCircuit/ForFPGA/mul_Dot Product11_dotp_15 ==
  In1 : Inport
  In2 : Inport  Port=2
  mul_Dot Product11_dotp_15 : Product  Inputs=**  OutDataTypeStr=single  SampleTime=6.02409638554217e-09
  mul_Dot Product11_dotp_15_pd1 : Delay  DelayLength=6
  Out1 : Outport
  wires:
  In1/1 -> mul_Dot Product11_dotp_15/1
  In2/1 -> mul_Dot Product11_dotp_15/2
  mul_Dot Product11_dotp_15/1 -> mul_Dot Product11_dotp_15_pd1/1
  mul_Dot Product11_dotp_15_pd1/1 -> Out1/1

== system gm_MATE_HDLsolver_myFirstCircuit/ForFPGA/mul_Dot Product11_dotp_2 ==
  In1 : Inport
  In2 : Inport  Port=2
  mul_Dot Product11_dotp_2 : Product  Inputs=**  OutDataTypeStr=single  SampleTime=6.02409638554217e-09
  mul_Dot Product11_dotp_2_pd1 : Delay  DelayLength=6
  Out1 : Outport
  wires:
  In1/1 -> mul_Dot Product11_dotp_2/1
  In2/1 -> mul_Dot Product11_dotp_2/2
  mul_Dot Product11_dotp_2/1 -> mul_Dot Product11_dotp_2_pd1/1
  mul_Dot Product11_dotp_2_pd1/1 -> Out1/1

== system gm_MATE_HDLsolver_myFirstCircuit/ForFPGA/mul_Dot Product11_dotp_3 ==
  In1 : Inport
  In2 : Inport  Port=2
  mul_Dot Product11_dotp_3 : Product  Inputs=**  OutDataTypeStr=single  SampleTime=6.02409638554217e-09
  mul_Dot Product11_dotp_3_pd1 : Delay  DelayLength=6
  Out1 : Outport
  wires:
  In1/1 -> mul_Dot Product11_dotp_3/1
  In2/1 -> mul_Dot Product11_dotp_3/2
  mul_Dot Product11_dotp_3/1 -> mul_Dot Product11_dotp_3_pd1/1
  mul_Dot Product11_dotp_3_pd1/1 -> Out1/1

== system gm_MATE_HDLsolver_myFirstCircuit/ForFPGA/mul_Dot Product11_dotp_4 ==
  In1 : Inport
  In2 : Inport  Port=2
  mul_Dot Product11_dotp_4 : Product  Inputs=**  OutDataTypeStr=single  SampleTime=6.02409638554217e-09
  mul_Dot Product11_dotp_4_pd1 : Delay  DelayLength=6
  Out1 : Outport
  wires:
  In1/1 -> mul_Dot Product11_dotp_4/1
  In2/1 -> mul_Dot Product11_dotp_4/2
  mul_Dot Product11_dotp_4/1 -> mul_Dot Product11_dotp_4_pd1/1
  mul_Dot Product11_dotp_4_pd1/1 -> Out1/1

== system gm_MATE_HDLsolver_myFirstCircuit/ForFPGA/mul_Dot Product11_dotp_5 ==
  In1 : Inport
  In2 : Inport  Port=2
  mul_Dot Product11_dotp_5 : Product  Inputs=**  OutDataTypeStr=single  SampleTime=6.02409638554217e-09
  mul_Dot Product11_dotp_5_pd1 : Delay  DelayLength=6
  Out1 : Outport
  wires:
  In1/1 -> mul_Dot Product11_dotp_5/1
  In2/1 -> mul_Dot Product11_dotp_5/2
  mul_Dot Product11_dotp_5/1 -> mul_Dot Product11_dotp_5_pd1/1
  mul_Dot Product11_dotp_5_pd1/1 -> Out1/1

== system gm_MATE_HDLsolver_myFirstCircuit/ForFPGA/mul_Dot Product11_dotp_6 ==
  In1 : Inport
  In2 : Inport  Port=2
  mul_Dot Product11_dotp_6 : Product  Inputs=**  OutDataTypeStr=single  SampleTime=6.02409638554217e-09
  mul_Dot Product11_dotp_6_pd1 : Delay  DelayLength=6
  Out1 : Outport
  wires:
  In1/1 -> mul_Dot Product11_dotp_6/1
  In2/1 -> mul_Dot Product11_dotp_6/2
  mul_Dot Product11_dotp_6/1 -> mul_Dot Product11_dotp_6_pd1/1
  mul_Dot Product11_dotp_6_pd1/1 -> Out1/1

== system gm_MATE_HDLsolver_myFirstCircuit/ForFPGA/mul_Dot Product11_dotp_7 ==
  In1 : Inport
  In2 : Inport  Port=2
  mul_Dot Product11_dotp_7 : Product  Inputs=**  OutDataTypeStr=single  SampleTime=6.02409638554217e-09
  mul_Dot Product11_dotp_7_pd1 : Delay  DelayLength=6
  Out1 : Outport
  wires:
  In1/1 -> mul_Dot Product11_dotp_7/1
  In2/1 -> mul_Dot Product11_dotp_7/2
  mul_Dot Product11_dotp_7/1 -> mul_Dot Product11_dotp_7_pd1/1
  mul_Dot Product11_dotp_7_pd1/1 -> Out1/1

== system gm_MATE_HDLsolver_myFirstCircuit/ForFPGA/mul_Dot Product11_dotp_8 ==
  In1 : Inport
  In2 : Inport  Port=2
  mul_Dot Product11_dotp_8 : Product  Inputs=**  OutDataTypeStr=single  SampleTime=6.02409638554217e-09
  mul_Dot Product11_dotp_8_pd1 : Delay  DelayLength=6
  Out1 : Outport
  wires:
  In1/1 -> mul_Dot Product11_dotp_8/1
  In2/1 -> mul_Dot Product11_dotp_8/2
  mul_Dot Product11_dotp_8/1 -> mul_Dot Product11_dotp_8_pd1/1
  mul_Dot Product11_dotp_8_pd1/1 -> Out1/1

== system gm_MATE_HDLsolver_myFirstCircuit/ForFPGA/mul_Dot Product11_dotp_9 ==
  In1 : Inport
  In2 : Inport  Port=2
  mul_Dot Product11_dotp_9 : Product  Inputs=**  OutDataTypeStr=single  SampleTime=6.02409638554217e-09
  mul_Dot Product11_dotp_9_pd1 : Delay  DelayLength=6
  Out1 : Outport
  wires:
  In1/1 -> mul_Dot Product11_dotp_9/1
  In2/1 -> mul_Dot Product11_dotp_9/2
  mul_Dot Product11_dotp_9/1 -> mul_Dot Product11_dotp_9_pd1/1
  mul_Dot Product11_dotp_9_pd1/1 -> Out1/1

== system gm_MATE_HDLsolver_myFirstCircuit/ForFPGA/mul_Dot Product12_dotp_0 ==
  In1 : Inport
  In2 : Inport  Port=2
  mul_Dot Product12_dotp_0 : Product  Inputs=**  OutDataTypeStr=single  SampleTime=6.02409638554217e-09
  mul_Dot Product12_dotp_0_pd1 : Delay  DelayLength=6
  Out1 : Outport
  wires:
  In1/1 -> mul_Dot Product12_dotp_0/1
  In2/1 -> mul_Dot Product12_dotp_0/2
  mul_Dot Product12_dotp_0/1 -> mul_Dot Product12_dotp_0_pd1/1
  mul_Dot Product12_dotp_0_pd1/1 -> Out1/1

== system gm_MATE_HDLsolver_myFirstCircuit/ForFPGA/mul_Dot Product12_dotp_1 ==
  In1 : Inport
  In2 : Inport  Port=2
  mul_Dot Product12_dotp_1 : Product  Inputs=**  OutDataTypeStr=single  SampleTime=6.02409638554217e-09
  mul_Dot Product12_dotp_1_pd1 : Delay  DelayLength=6
  Out1 : Outport
  wires:
  In1/1 -> mul_Dot Product12_dotp_1/1
  In2/1 -> mul_Dot Product12_dotp_1/2
  mul_Dot Product12_dotp_1/1 -> mul_Dot Product12_dotp_1_pd1/1
  mul_Dot Product12_dotp_1_pd1/1 -> Out1/1

== system gm_MATE_HDLsolver_myFirstCircuit/ForFPGA/mul_Dot Product12_dotp_10 ==
  In1 : Inport
  In2 : Inport  Port=2
  mul_Dot Product12_dotp_10 : Product  Inputs=**  OutDataTypeStr=single  SampleTime=6.02409638554217e-09
  mul_Dot Product12_dotp_10_pd1 : Delay  DelayLength=6
  Out1 : Outport
  wires:
  In1/1 -> mul_Dot Product12_dotp_10/1
  In2/1 -> mul_Dot Product12_dotp_10/2
  mul_Dot Product12_dotp_10/1 -> mul_Dot Product12_dotp_10_pd1/1
  mul_Dot Product12_dotp_10_pd1/1 -> Out1/1

== system gm_MATE_HDLsolver_myFirstCircuit/ForFPGA/mul_Dot Product12_dotp_11 ==
  In1 : Inport
  In2 : Inport  Port=2
  mul_Dot Product12_dotp_11 : Product  Inputs=**  OutDataTypeStr=single  SampleTime=6.02409638554217e-09
  mul_Dot Product12_dotp_11_pd1 : Delay  DelayLength=6
  Out1 : Outport
  wires:
  In1/1 -> mul_Dot Product12_dotp_11/1
  In2/1 -> mul_Dot Product12_dotp_11/2
  mul_Dot Product12_dotp_11/1 -> mul_Dot Product12_dotp_11_pd1/1
  mul_Dot Product12_dotp_11_pd1/1 -> Out1/1

== system gm_MATE_HDLsolver_myFirstCircuit/ForFPGA/mul_Dot Product12_dotp_12 ==
  In1 : Inport
  In2 : Inport  Port=2
  mul_Dot Product12_dotp_12 : Product  Inputs=**  OutDataTypeStr=single  SampleTime=6.02409638554217e-09
  mul_Dot Product12_dotp_12_pd1 : Delay  DelayLength=6
  Out1 : Outport
  wires:
  In1/1 -> mul_Dot Product12_dotp_12/1
  In2/1 -> mul_Dot Product12_dotp_12/2
  mul_Dot Product12_dotp_12/1 -> mul_Dot Product12_dotp_12_pd1/1
  mul_Dot Product12_dotp_12_pd1/1 -> Out1/1

== system gm_MATE_HDLsolver_myFirstCircuit/ForFPGA/mul_Dot Product12_dotp_13 ==
  In1 : Inport
  In2 : Inport  Port=2
  mul_Dot Product12_dotp_13 : Product  Inputs=**  OutDataTypeStr=single  SampleTime=6.02409638554217e-09
  mul_Dot Product12_dotp_13_pd1 : Delay  DelayLength=6
  Out1 : Outport
  wires:
  In1/1 -> mul_Dot Product12_dotp_13/1
  In2/1 -> mul_Dot Product12_dotp_13/2
  mul_Dot Product12_dotp_13/1 -> mul_Dot Product12_dotp_13_pd1/1
  mul_Dot Product12_dotp_13_pd1/1 -> Out1/1

== system gm_MATE_HDLsolver_myFirstCircuit/ForFPGA/mul_Dot Product12_dotp_14 ==
  In1 : Inport
  In2 : Inport  Port=2
  mul_Dot Product12_dotp_14 : Product  Inputs=**  OutDataTypeStr=single  SampleTime=6.02409638554217e-09
  mul_Dot Product12_dotp_14_pd1 : Delay  DelayLength=6
  Out1 : Outport
  wires:
  In1/1 -> mul_Dot Product12_dotp_14/1
  In2/1 -> mul_Dot Product12_dotp_14/2
  mul_Dot Product12_dotp_14/1 -> mul_Dot Product12_dotp_14_pd1/1
  mul_Dot Product12_dotp_14_pd1/1 -> Out1/1

== system gm_MATE_HDLsolver_myFirstCircuit/ForFPGA/mul_Dot Product12_dotp_15 ==
  In1 : Inport
  In2 : Inport  Port=2
  mul_Dot Product12_dotp_15 : Product  Inputs=**  OutDataTypeStr=single  SampleTime=6.02409638554217e-09
  mul_Dot Product12_dotp_15_pd1 : Delay  DelayLength=6
  Out1 : Outport
  wires:
  In1/1 -> mul_Dot Product12_dotp_15/1
  In2/1 -> mul_Dot Product12_dotp_15/2
  mul_Dot Product12_dotp_15/1 -> mul_Dot Product12_dotp_15_pd1/1
  mul_Dot Product12_dotp_15_pd1/1 -> Out1/1

== system gm_MATE_HDLsolver_myFirstCircuit/ForFPGA/mul_Dot Product12_dotp_2 ==
  In1 : Inport
  In2 : Inport  Port=2
  mul_Dot Product12_dotp_2 : Product  Inputs=**  OutDataTypeStr=single  SampleTime=6.02409638554217e-09
  mul_Dot Product12_dotp_2_pd1 : Delay  DelayLength=6
  Out1 : Outport
  wires:
  In1/1 -> mul_Dot Product12_dotp_2/1
  In2/1 -> mul_Dot Product12_dotp_2/2
  mul_Dot Product12_dotp_2/1 -> mul_Dot Product12_dotp_2_pd1/1
  mul_Dot Product12_dotp_2_pd1/1 -> Out1/1

== system gm_MATE_HDLsolver_myFirstCircuit/ForFPGA/mul_Dot Product12_dotp_3 ==
  In1 : Inport
  In2 : Inport  Port=2
  mul_Dot Product12_dotp_3 : Product  Inputs=**  OutDataTypeStr=single  SampleTime=6.02409638554217e-09
  mul_Dot Product12_dotp_3_pd1 : Delay  DelayLength=6
  Out1 : Outport
  wires:
  In1/1 -> mul_Dot Product12_dotp_3/1
  In2/1 -> mul_Dot Product12_dotp_3/2
  mul_Dot Product12_dotp_3/1 -> mul_Dot Product12_dotp_3_pd1/1
  mul_Dot Product12_dotp_3_pd1/1 -> Out1/1

== system gm_MATE_HDLsolver_myFirstCircuit/ForFPGA/mul_Dot Product12_dotp_4 ==
  In1 : Inport
  In2 : Inport  Port=2
  mul_Dot Product12_dotp_4 : Product  Inputs=**  OutDataTypeStr=single  SampleTime=6.02409638554217e-09
  mul_Dot Product12_dotp_4_pd1 : Delay  DelayLength=6
  Out1 : Outport
  wires:
  In1/1 -> mul_Dot Product12_dotp_4/1
  In2/1 -> mul_Dot Product12_dotp_4/2
  mul_Dot Product12_dotp_4/1 -> mul_Dot Product12_dotp_4_pd1/1
  mul_Dot Product12_dotp_4_pd1/1 -> Out1/1

== system gm_MATE_HDLsolver_myFirstCircuit/ForFPGA/mul_Dot Product12_dotp_5 ==
  In1 : Inport
  In2 : Inport  Port=2
  mul_Dot Product12_dotp_5 : Product  Inputs=**  OutDataTypeStr=single  SampleTime=6.02409638554217e-09
  mul_Dot Product12_dotp_5_pd1 : Delay  DelayLength=6
  Out1 : Outport
  wires:
  In1/1 -> mul_Dot Product12_dotp_5/1
  In2/1 -> mul_Dot Product12_dotp_5/2
  mul_Dot Product12_dotp_5/1 -> mul_Dot Product12_dotp_5_pd1/1
  mul_Dot Product12_dotp_5_pd1/1 -> Out1/1

== system gm_MATE_HDLsolver_myFirstCircuit/ForFPGA/mul_Dot Product12_dotp_6 ==
  In1 : Inport
  In2 : Inport  Port=2
  mul_Dot Product12_dotp_6 : Product  Inputs=**  OutDataTypeStr=single  SampleTime=6.02409638554217e-09
  mul_Dot Product12_dotp_6_pd1 : Delay  DelayLength=6
  Out1 : Outport
  wires:
  In1/1 -> mul_Dot Product12_dotp_6/1
  In2/1 -> mul_Dot Product12_dotp_6/2
  mul_Dot Product12_dotp_6/1 -> mul_Dot Product12_dotp_6_pd1/1
  mul_Dot Product12_dotp_6_pd1/1 -> Out1/1

== system gm_MATE_HDLsolver_myFirstCircuit/ForFPGA/mul_Dot Product12_dotp_7 ==
  In1 : Inport
  In2 : Inport  Port=2
  mul_Dot Product12_dotp_7 : Product  Inputs=**  OutDataTypeStr=single  SampleTime=6.02409638554217e-09
  mul_Dot Product12_dotp_7_pd1 : Delay  DelayLength=6
  Out1 : Outport
  wires:
  In1/1 -> mul_Dot Product12_dotp_7/1
  In2/1 -> mul_Dot Product12_dotp_7/2
  mul_Dot Product12_dotp_7/1 -> mul_Dot Product12_dotp_7_pd1/1
  mul_Dot Product12_dotp_7_pd1/1 -> Out1/1

== system gm_MATE_HDLsolver_myFirstCircuit/ForFPGA/mul_Dot Product12_dotp_8 ==
  In1 : Inport
  In2 : Inport  Port=2
  mul_Dot Product12_dotp_8 : Product  Inputs=**  OutDataTypeStr=single  SampleTime=6.02409638554217e-09
  mul_Dot Product12_dotp_8_pd1 : Delay  DelayLength=6
  Out1 : Outport
  wires:
  In1/1 -> mul_Dot Product12_dotp_8/1
  In2/1 -> mul_Dot Product12_dotp_8/2
  mul_Dot Product12_dotp_8/1 -> mul_Dot Product12_dotp_8_pd1/1
  mul_Dot Product12_dotp_8_pd1/1 -> Out1/1

== system gm_MATE_HDLsolver_myFirstCircuit/ForFPGA/mul_Dot Product12_dotp_9 ==
  In1 : Inport
  In2 : Inport  Port=2
  mul_Dot Product12_dotp_9 : Product  Inputs=**  OutDataTypeStr=single  SampleTime=6.02409638554217e-09
  mul_Dot Product12_dotp_9_pd1 : Delay  DelayLength=6
  Out1 : Outport
  wires:
  In1/1 -> mul_Dot Product12_dotp_9/1
  In2/1 -> mul_Dot Product12_dotp_9/2
  mul_Dot Product12_dotp_9/1 -> mul_Dot Product12_dotp_9_pd1/1
  mul_Dot Product12_dotp_9_pd1/1 -> Out1/1

== system gm_MATE_HDLsolver_myFirstCircuit/ForFPGA/mul_Dot Product13_dotp_0 ==
  In1 : Inport
  In2 : Inport  Port=2
  mul_Dot Product13_dotp_0 : Product  Inputs=**  OutDataTypeStr=single  SampleTime=6.02409638554217e-09
  mul_Dot Product13_dotp_0_pd1 : Delay  DelayLength=6
  Out1 : Outport
  wires:
  In1/1 -> mul_Dot Product13_dotp_0/1
  In2/1 -> mul_Dot Product13_dotp_0/2
  mul_Dot Product13_dotp_0/1 -> mul_Dot Product13_dotp_0_pd1/1
  mul_Dot Product13_dotp_0_pd1/1 -> Out1/1

== system gm_MATE_HDLsolver_myFirstCircuit/ForFPGA/mul_Dot Product13_dotp_1 ==
  In1 : Inport
  In2 : Inport  Port=2
  mul_Dot Product13_dotp_1 : Product  Inputs=**  OutDataTypeStr=single  SampleTime=6.02409638554217e-09
  mul_Dot Product13_dotp_1_pd1 : Delay  DelayLength=6
  Out1 : Outport
  wires:
  In1/1 -> mul_Dot Product13_dotp_1/1
  In2/1 -> mul_Dot Product13_dotp_1/2
  mul_Dot Product13_dotp_1/1 -> mul_Dot Product13_dotp_1_pd1/1
  mul_Dot Product13_dotp_1_pd1/1 -> Out1/1

== system gm_MATE_HDLsolver_myFirstCircuit/ForFPGA/mul_Dot Product13_dotp_10 ==
  In1 : Inport
  In2 : Inport  Port=2
  mul_Dot Product13_dotp_10 : Product  Inputs=**  OutDataTypeStr=single  SampleTime=6.02409638554217e-09
  mul_Dot Product13_dotp_10_pd1 : Delay  DelayLength=6
  Out1 : Outport
  wires:
  In1/1 -> mul_Dot Product13_dotp_10/1
  In2/1 -> mul_Dot Product13_dotp_10/2
  mul_Dot Product13_dotp_10/1 -> mul_Dot Product13_dotp_10_pd1/1
  mul_Dot Product13_dotp_10_pd1/1 -> Out1/1

== system gm_MATE_HDLsolver_myFirstCircuit/ForFPGA/mul_Dot Product13_dotp_11 ==
  In1 : Inport
  In2 : Inport  Port=2
  mul_Dot Product13_dotp_11 : Product  Inputs=**  OutDataTypeStr=single  SampleTime=6.02409638554217e-09
  mul_Dot Product13_dotp_11_pd1 : Delay  DelayLength=6
  Out1 : Outport
  wires:
  In1/1 -> mul_Dot Product13_dotp_11/1
  In2/1 -> mul_Dot Product13_dotp_11/2
  mul_Dot Product13_dotp_11/1 -> mul_Dot Product13_dotp_11_pd1/1
  mul_Dot Product13_dotp_11_pd1/1 -> Out1/1

== system gm_MATE_HDLsolver_myFirstCircuit/ForFPGA/mul_Dot Product13_dotp_12 ==
  In1 : Inport
  In2 : Inport  Port=2
  mul_Dot Product13_dotp_12 : Product  Inputs=**  OutDataTypeStr=single  SampleTime=6.02409638554217e-09
  mul_Dot Product13_dotp_12_pd1 : Delay  DelayLength=6
  Out1 : Outport
  wires:
  In1/1 -> mul_Dot Product13_dotp_12/1
  In2/1 -> mul_Dot Product13_dotp_12/2
  mul_Dot Product13_dotp_12/1 -> mul_Dot Product13_dotp_12_pd1/1
  mul_Dot Product13_dotp_12_pd1/1 -> Out1/1

== system gm_MATE_HDLsolver_myFirstCircuit/ForFPGA/mul_Dot Product13_dotp_13 ==
  In1 : Inport
  In2 : Inport  Port=2
  mul_Dot Product13_dotp_13 : Product  Inputs=**  OutDataTypeStr=single  SampleTime=6.02409638554217e-09
  mul_Dot Product13_dotp_13_pd1 : Delay  DelayLength=6
  Out1 : Outport
  wires:
  In1/1 -> mul_Dot Product13_dotp_13/1
  In2/1 -> mul_Dot Product13_dotp_13/2
  mul_Dot Product13_dotp_13/1 -> mul_Dot Product13_dotp_13_pd1/1
  mul_Dot Product13_dotp_13_pd1/1 -> Out1/1

== system gm_MATE_HDLsolver_myFirstCircuit/ForFPGA/mul_Dot Product13_dotp_14 ==
  In1 : Inport
  In2 : Inport  Port=2
  mul_Dot Product13_dotp_14 : Product  Inputs=**  OutDataTypeStr=single  SampleTime=6.02409638554217e-09
  mul_Dot Product13_dotp_14_pd1 : Delay  DelayLength=6
  Out1 : Outport
  wires:
  In1/1 -> mul_Dot Product13_dotp_14/1
  In2/1 -> mul_Dot Product13_dotp_14/2
  mul_Dot Product13_dotp_14/1 -> mul_Dot Product13_dotp_14_pd1/1
  mul_Dot Product13_dotp_14_pd1/1 -> Out1/1

== system gm_MATE_HDLsolver_myFirstCircuit/ForFPGA/mul_Dot Product13_dotp_15 ==
  In1 : Inport
  In2 : Inport  Port=2
  mul_Dot Product13_dotp_15 : Product  Inputs=**  OutDataTypeStr=single  SampleTime=6.02409638554217e-09
  mul_Dot Product13_dotp_15_pd1 : Delay  DelayLength=6
  Out1 : Outport
  wires:
  In1/1 -> mul_Dot Product13_dotp_15/1
  In2/1 -> mul_Dot Product13_dotp_15/2
  mul_Dot Product13_dotp_15/1 -> mul_Dot Product13_dotp_15_pd1/1
  mul_Dot Product13_dotp_15_pd1/1 -> Out1/1

== system gm_MATE_HDLsolver_myFirstCircuit/ForFPGA/mul_Dot Product13_dotp_2 ==
  In1 : Inport
  In2 : Inport  Port=2
  mul_Dot Product13_dotp_2 : Product  Inputs=**  OutDataTypeStr=single  SampleTime=6.02409638554217e-09
  mul_Dot Product13_dotp_2_pd1 : Delay  DelayLength=6
  Out1 : Outport
  wires:
  In1/1 -> mul_Dot Product13_dotp_2/1
  In2/1 -> mul_Dot Product13_dotp_2/2
  mul_Dot Product13_dotp_2/1 -> mul_Dot Product13_dotp_2_pd1/1
  mul_Dot Product13_dotp_2_pd1/1 -> Out1/1

== system gm_MATE_HDLsolver_myFirstCircuit/ForFPGA/mul_Dot Product13_dotp_3 ==
  In1 : Inport
  In2 : Inport  Port=2
  mul_Dot Product13_dotp_3 : Product  Inputs=**  OutDataTypeStr=single  SampleTime=6.02409638554217e-09
  mul_Dot Product13_dotp_3_pd1 : Delay  DelayLength=6
  Out1 : Outport
  wires:
  In1/1 -> mul_Dot Product13_dotp_3/1
  In2/1 -> mul_Dot Product13_dotp_3/2
  mul_Dot Product13_dotp_3/1 -> mul_Dot Product13_dotp_3_pd1/1
  mul_Dot Product13_dotp_3_pd1/1 -> Out1/1

== system gm_MATE_HDLsolver_myFirstCircuit/ForFPGA/mul_Dot Product13_dotp_4 ==
  In1 : Inport
  In2 : Inport  Port=2
  mul_Dot Product13_dotp_4 : Product  Inputs=**  OutDataTypeStr=single  SampleTime=6.02409638554217e-09
  mul_Dot Product13_dotp_4_pd1 : Delay  DelayLength=6
  Out1 : Outport
  wires:
  In1/1 -> mul_Dot Product13_dotp_4/1
  In2/1 -> mul_Dot Product13_dotp_4/2
  mul_Dot Product13_dotp_4/1 -> mul_Dot Product13_dotp_4_pd1/1
  mul_Dot Product13_dotp_4_pd1/1 -> Out1/1

== system gm_MATE_HDLsolver_myFirstCircuit/ForFPGA/mul_Dot Product13_dotp_5 ==
  In1 : Inport
  In2 : Inport  Port=2
  mul_Dot Product13_dotp_5 : Product  Inputs=**  OutDataTypeStr=single  SampleTime=6.02409638554217e-09
  mul_Dot Product13_dotp_5_pd1 : Delay  DelayLength=6
  Out1 : Outport
  wires:
  In1/1 -> mul_Dot Product13_dotp_5/1
  In2/1 -> mul_Dot Product13_dotp_5/2
  mul_Dot Product13_dotp_5/1 -> mul_Dot Product13_dotp_5_pd1/1
  mul_Dot Product13_dotp_5_pd1/1 -> Out1/1

== system gm_MATE_HDLsolver_myFirstCircuit/ForFPGA/mul_Dot Product13_dotp_6 ==
  In1 : Inport
  In2 : Inport  Port=2
  mul_Dot Product13_dotp_6 : Product  Inputs=**  OutDataTypeStr=single  SampleTime=6.02409638554217e-09
  mul_Dot Product13_dotp_6_pd1 : Delay  DelayLength=6
  Out1 : Outport
  wires:
  In1/1 -> mul_Dot Product13_dotp_6/1
  In2/1 -> mul_Dot Product13_dotp_6/2
  mul_Dot Product13_dotp_6/1 -> mul_Dot Product13_dotp_6_pd1/1
  mul_Dot Product13_dotp_6_pd1/1 -> Out1/1
